simulink model "diff1"  (R2021a)
settings: Solver=VariableStepAuto  StartTime=0.0  StopTime=10.0  RelTol=1e-3
undefined symbols (not defined in the file): PI
libraries: simulink x1
settings Model: Creator=Oleg  LastModifiedBy=Oleg

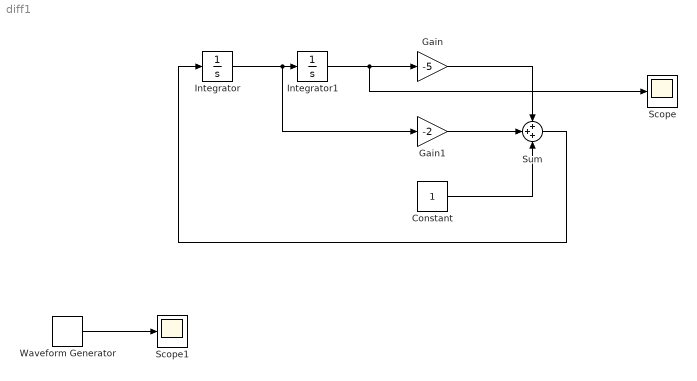
== system diff1 ==
  Constant : Constant
  Gain : Gain  Gain=-5
  Gain1 : Gain  Gain=-2
  Integrator : Integrator
  Integrator1 : Integrator
  Scope : Scope
  Scope1 : Scope
  Sum : Sum  Inputs=+++
  Waveform Generator : simulink/Sources/Waveform Generator  OutMin=[]  OutMax=[]  OutDataTypeStr=double  SelectedSignal=1  Signals=sin(1,2*PI*4,0)  BlockNames=MultiportSwitch_7206b278474d4fd  SampleTime=0.001
  wires:
  Gain/1 -> Sum/1
  Gain1/1 -> Sum/2
  Constant/1 -> Sum/3
  Integrator1/1 -> Scope/1, Gain/1
  Integrator/1 -> Gain1/1, Integrator1/1
  Sum/1 -> Integrator/1
  Waveform Generator/1 -> Scope1/1
